simulink model "hybrid_photovoltaic_wind_power_sysytem_grid"  (R2024b)
settings: Solver=ode45  StartTime=0.0  StopTime=1  RelTol=1e-3  EnableMultiTasking=on
undefined symbols (not defined in the file): DiscIntNeverNeededParam, find_system
libraries: powerlib_extras x39, spsThreePhaseVIMeasurementLib x12, spsSeriesRLCBranchLib x5, spsDiodeLib x4, spsUniversalBridgeLib x4, simulink_extras x4, spsThreePhaseBreakerLib x3, spsLoadFlowBusLib x3, spsVoltageMeasurementLib x2, slpidlib x2, spsThreePhaseSeriesRLCLoadLib x2, spsThreePhaseTransformerInductanceMatrixTypeTwoWindingsLib x2
(part 2 of 4)

== system hybrid_photovoltaic_wind_power_sysytem_grid/Hybrid Photovoltaic and Wind power system/VSC1 Control/Current Regulator ==
  note: For Ltot >> Rtot :
  note: (Vq_prim - Vq_conv) ~ = - Id * Ltot
  note: (Vd_prim - Vd_conv) ~= + Iq * Ltot
  note: Ltot = Lxfo + Lchoke
      | Rtot = Rxfo + Rchoke
  note: Id positive --> The converter generates active power ("Inverter mode") = Active Power P positive
  note: Iq positive --> The converter absorbs reactive power ("Inductive mode") = Reactive Power Q negative
  note: Sign Convention: Current going out of the converter = positive current
  note: Current Regulator
      | (with feedforward)
  note: Vq_mes + Id*L + Iq*R + deriv(Iq)*L= Vq_conv
  note: Vd_mes + Id*R - Iq*L + deriv(Id)*L= Vd_conv
  note: harmonic filter neglected
  VdVq_mes : Inport  PortDimensions=2
  IdIq_mes : Inport  Port=2  PortDimensions=2
  IdIq_ref : Inport  Port=3  PortDimensions=2
  Add1 : Sum  Inputs=++-
  Add2 : Sum
  Add3 : Sum  Inputs=+++
  Demux : Demux  Outputs=2
  Demux1 : Demux  Outputs=2
  Ltot_pu1 : Gain  Gain=Ltot_pu  SaturateOnIntegerOverflow=on  OutDataTypeStr=Inherit: Same as input  ParamDataTypeStr=Inherit: Same as input
  Ltot_pu2 : Gain  Gain=Ltot_pu  SaturateOnIntegerOverflow=on  OutDataTypeStr=Inherit: Same as input  ParamDataTypeStr=Inherit: Same as input
  Mux : Mux  Inputs=2
  PI : slpidlib/PID Controller  Controller=PI  Form=Parallel  TimeDomain=Discrete-time  UseExternalTs=off  SampleTime=Ts  IntegratorMethod=Forward Euler  FilterMethod=Forward Euler  ControllerParametersSource=internal  P=Kp_Ireg  I=Ki_Ireg  UseKiTs=off  D=0  UseExternalDerivativeSource=off  N=100  UseFilter=on  TunerSelectOption=Transfer Function Based (PID Tuner App)  InitialConditionSource=internal  InitialConditionForIntegrator=0  InitialConditionForFilter=0  DifferentiatorICPrevScaledInput=0  ExternalReset=none  TrackingMode=off  Kt=1  LimitOutput=on  SatLimitsSource=internal  UpperSaturationLimit=2  LowerSaturationLimit=-2  LinearizeAsGain=off  AntiWindupMode=none  Kb=1  LimitIntegrator=off  UpperIntegratorSaturationLimit=inf  LowerIntegratorSaturationLimit=-inf  POutMin=[]  POutMax=[]  IOutMin=[]  IOutMax=[]  DOutMin=[]  DOutMax=[]  NOutMin=[]  NOutMax=[]  SumOutMin=[]  SumOutMax=[]  SaturationOutMin=[]  SaturationOutMax=[]  PParamMin=[]  PParamMax=[]  IParamMin=[]  IParamMax=[]  DParamMin=[]  DParamMax=[]  NParamMin=[]  NParamMax=[]  KbParamMin=[]  KbParamMax=[]  KtParamMin=[]  KtParamMax=[]  KbOutMin=[]  KbOutMax=[]  KtOutMin=[]  KtOutMax=[]  IntegratorOutMin=[]  IntegratorOutMax=[]  FilterOutMin=[]  FilterOutMax=[]  SumI1OutMin=[]  SumI1OutMax=[]  SumI2OutMin=[]  SumI2OutMax=[]  SumI3OutMin=[]  SumI3OutMax=[]  SumI4OutMin=[]  SumI4OutMax=[]  SumDOutMin=[]  SumDOutMax=[]  DifferentiatorOutMin=[]  DifferentiatorOutMax=[]  FilterDiffOutCoefMin=[]  FilterDiffOutCoefMax=[]  ReciprocalOutMin=[]  ReciprocalOutMax=[]  SumDenOutMin=[]  SumDenOutMax=[]  SumNumOutMin=[]  SumNumOutMax=[]  DivideOutMin=[]  DivideOutMax=[]  UdiffTsProdOutMin=[]  UdiffTsProdOutMax=[]  NTsProdOutMin=[]  NTsProdOutMax=[]  UintegralTsProdOutMin=[]  UintegralTsProdOutMax=[]  UngainTsProdOutMin=[]  UngainTsProdOutMax=[]  ClampingZeroOutDataTypeStr=Inherit: Inherit via back propagation  ClampingZeroOutMin=[]  ClampingZeroOutMax=[]  FilterDenConstantOutDataTypeStr=Inherit: Inherit via back propagation  FilterDenConstantOutMin=[]  FilterDenConstantOutMax=[]  PCopyOutDataTypeStr=Inherit: Inherit via back propagation  PCopyOutMin=[]  PCopyOutMax=[]  NCopyOutDataTypeStr=Inherit: Inherit via back propagation  NCopyOutMin=[]  NCopyOutMax=[]  IntegratorContinuousStateAttributes=''  IntegratorStateMustResolveToSignalObject=off  IntegratorRTWStateStorageClass=Auto  FilterContinuousStateAttributes=''  FilterStateMustResolveToSignalObject=off  FilterRTWStateStorageClass=Auto  ParallelPVariant=InternalParameters  IdealPVariant=Disabled  IVariant=InternalParameters  DVariant=Disabled  IntegratorVariant=Discrete  SatVariant=Enabled  AWVariant=Passthrough  PCopyVariant=Disabled  TRVariant=Disabled  FdbkBlocksVariant=Forward  IdealPFdbkVariant=Disabled  SatFdbkVariant=Disabled  DerivativeFilterVariant=Disabled  NVariant=Disabled  NCopyVariant=Disabled_SignalSpec  FilterICVariant=Disabled  IntegratorICVariant=InternalICs  ExternalResetVariant=Disabled  TRSumVariant=Passthrough  SumFdbkVariant=Disabled  SumVariant=Sum_PI  TsampFilterVariant=InternalTs  TsampNgainVariant=Passthrough  TsampIntegralVariant=Disabled_SignalSpec  ExternalSaturationOutDataTypeStr=Inherit: Same as second input  DerivativeSourceVariant=Disabled  PreIntVariant=InternalPreInt
  PI_Ireg1 : Scope
  Rtot_pu1 : Gain  Gain=Rtot_pu  SaturateOnIntegerOverflow=on  OutDataTypeStr=Inherit: Same as input  ParamDataTypeStr=Inherit: Same as input
  Rtot_pu5 : Gain  Gain=Rtot_pu  SaturateOnIntegerOverflow=on  OutDataTypeStr=Inherit: Same as input  ParamDataTypeStr=Inherit: Same as input
  Saturation : Saturate  UpperLimit=2  LowerLimit=-2
  Sum : Sum  Inputs=|-+
  VdVq_conv : Outport
  wires:
  Add3/1 -> Mux/2
  Demux/2 -> Add3/1
  Add1/1 -> Mux/1  "Feedforward"
  Ltot_pu2/1 -> Add3/3
  Rtot_pu5/1 -> Add3/2
  Demux1/2 -> Rtot_pu5/1, Ltot_pu1/1
  Ltot_pu1/1 -> Add1/3
  Demux1/1 -> Ltot_pu2/1, Rtot_pu1/1
  Rtot_pu1/1 -> Add1/2
  Demux/1 -> Add1/1
  VdVq_mes/1 -> Demux/1
  Saturation/1 -> VdVq_conv/1
  Add2/1 -> Saturation/1
  IdIq_mes/1 -> Sum/1
  IdIq_ref/1 -> Demux1/1, Sum/2
  Sum/1 -> PI/1
  PI/1 -> Add2/1  "PI"
  Mux/1 -> Add2/2, PI_Ireg1/1

== system hybrid_photovoltaic_wind_power_sysytem_grid/Hybrid Photovoltaic and Wind power system/VSC1 Control/PLL & Measurements ==
  Vabc_prim : Inport
  Iabc_prim : Inport  Port=2
  PLL : powerlib_extras/Discrete  Control Blocks/Discrete 3-phase PLL  Fmin=45  Par_Init="[-0.57  Fnom]"  ParK=[60 1400]  Ts=Ts  AGC=off
  Selector1 : Selector  InputPortWidth=3  IndexOptions=Index vector (dialog)  Indices=[1 2]  OutputSizes=1
  Selector2 : Selector  InputPortWidth=3  IndexOptions=Index vector (dialog)  Indices=[1 2]  OutputSizes=1
  Terminator : Terminator
  V->pu : Gain  Gain=1/(Vnom_prim*sqrt(2)/sqrt(3))  SaturateOnIntegerOverflow=on  OutDataTypeStr=Inherit: Same as input  ParamDataTypeStr=Inherit: Same as input
  V->pu1 : Gain  Gain=Vnom_prim*sqrt(3)/Pnom/sqrt(2)  SaturateOnIntegerOverflow=on  OutDataTypeStr=Inherit: Same as input  ParamDataTypeStr=Inherit: Same as input
  abc_to_dq0 Transformation1 : powerlib_extras/Measurements/abc_to_dq0 Transformation
  abc_to_dq0 Transformation2 : powerlib_extras/Measurements/abc_to_dq0 Transformation
  wt : Outport
  VdVq_prim : Outport  Port=2
  IdIq_prim : Outport  Port=3
  wires:
  PLL/1 -> Terminator/1
  PLL/3 -> abc_to_dq0 Transformation1/2, abc_to_dq0 Transformation2/2
  Selector1/1 -> IdIq_prim/1
  Selector2/1 -> VdVq_prim/1
  abc_to_dq0 Transformation1/1 -> Selector2/1
  Iabc_prim/1 -> V->pu1/1
  Vabc_prim/1 -> V->pu/1
  PLL/2 -> wt/1
  abc_to_dq0 Transformation2/1 -> Selector1/1
  V->pu/1 -> abc_to_dq0 Transformation1/1, PLL/1
  V->pu1/1 -> abc_to_dq0 Transformation2/1

== system hybrid_photovoltaic_wind_power_sysytem_grid/Hybrid Photovoltaic and Wind power system/VSC1 Control/Uabc_ref Generation max (m) = 1 ==
  note: (Correction for delai of Ts_Control)
  note: (Correction for transformer
      |  D1 connection)
  wt : Inport
  VdVq_conv : Inport  Port=2
  Add1 : Sum  Inputs=++++
  Add2 : Sum
  Complex to Magnitude-Angle : ComplexToMagnitudeAngle
  Constant : Constant  Value=-pi/6
  Constant1 : Constant  Value=Vnom_dc
  Constant2 : Constant  Value="[ 0  -2*pi/3  2*pi/3  ]"
  Constant3 : Constant  Value=Vnom_sec*sqrt(2)/sqrt(3)
  Constant4 : Constant  Value=Ts*Fnom*(2*pi)
  Demux1 : Demux  Outputs=2
  Gain1 : Gain  Gain=1/2
  Product : Product  Inputs=*/  RndMeth=Zero
  Product1 : Product  Inputs=*/  RndMeth=Zero
  Product2 : Product  Inputs=**  RndMeth=Zero
  Real-Imag to Complex : RealImagToComplex
  Saturation : Saturate  UpperLimit=1  LowerLimit=0
  Trigonometric Function : Trigonometry
  Uabc_ref : Outport
  tag scope: m=global
  wires:
  Constant4/1 -> Add1/4
  wt/1 -> Add1/1
  Product2/1 -> Uabc_ref/1
  Trigonometric Function/1 -> Product2/2
  Saturation/1 -> Product2/1, [m]
  Add2/1 -> Trigonometric Function/1
  Add1/1 -> Add2/2
  Complex to Magnitude-Angle/2 -> Add2/1
  Product/1 -> Product1/2
  Constant3/1 -> Product/2
  Constant/1 -> Add1/3
  Constant2/1 -> Add1/2
  Demux1/2 -> Real-Imag to Complex/2
  Demux1/1 -> Real-Imag to Complex/1
  Real-Imag to Complex/1 -> Complex to Magnitude-Angle/1
  Gain1/1 -> Product/1
  Product1/1 -> Demux1/1
  VdVq_conv/1 -> Product1/1
  Constant1/1 -> Gain1/1
  Complex to Magnitude-Angle/1 -> Saturation/1

== system hybrid_photovoltaic_wind_power_sysytem_grid/Hybrid Photovoltaic and Wind power system/VSC1 Control/VDC Regulator ==
  Vdc_mes : Inport  PortDimensions=1
  Vdc_ref : Inport  Port=2  PortDimensions=1
  PI : slpidlib/PID Controller  Controller=PI  Form=Parallel  TimeDomain=Discrete-time  UseExternalTs=off  SampleTime=Ts  IntegratorMethod=Trapezoidal  FilterMethod=Forward Euler  ControllerParametersSource=internal  P=Kp_VDCreg  I=Ki_VDCreg  UseKiTs=off  D=0  UseExternalDerivativeSource=off  N=100  UseFilter=on  TunerSelectOption=Transfer Function Based (PID Tuner App)  InitialConditionSource=internal  InitialConditionForIntegrator=0  InitialConditionForFilter=0  DifferentiatorICPrevScaledInput=0  ExternalReset=none  TrackingMode=off  Kt=1  LimitOutput=on  SatLimitsSource=internal  UpperSaturationLimit=1.5  LowerSaturationLimit=-1.5  LinearizeAsGain=off  AntiWindupMode=none  Kb=1  LimitIntegrator=off  UpperIntegratorSaturationLimit=inf  LowerIntegratorSaturationLimit=-inf  POutMin=[]  POutMax=[]  IOutMin=[]  IOutMax=[]  DOutMin=[]  DOutMax=[]  NOutMin=[]  NOutMax=[]  SumOutMin=[]  SumOutMax=[]  SaturationOutMin=[]  SaturationOutMax=[]  PParamMin=[]  PParamMax=[]  IParamMin=[]  IParamMax=[]  DParamMin=[]  DParamMax=[]  NParamMin=[]  NParamMax=[]  KbParamMin=[]  KbParamMax=[]  KtParamMin=[]  KtParamMax=[]  KbOutMin=[]  KbOutMax=[]  KtOutMin=[]  KtOutMax=[]  IntegratorOutMin=[]  IntegratorOutMax=[]  FilterOutMin=[]  FilterOutMax=[]  SumI1OutMin=[]  SumI1OutMax=[]  SumI2OutMin=[]  SumI2OutMax=[]  SumI3OutMin=[]  SumI3OutMax=[]  SumI4OutMin=[]  SumI4OutMax=[]  SumDOutMin=[]  SumDOutMax=[]  DifferentiatorOutMin=[]  DifferentiatorOutMax=[]  FilterDiffOutCoefMin=[]  FilterDiffOutCoefMax=[]  ReciprocalOutMin=[]  ReciprocalOutMax=[]  SumDenOutMin=[]  SumDenOutMax=[]  SumNumOutMin=[]  SumNumOutMax=[]  DivideOutMin=[]  DivideOutMax=[]  UdiffTsProdOutMin=[]  UdiffTsProdOutMax=[]  NTsProdOutMin=[]  NTsProdOutMax=[]  UintegralTsProdOutMin=[]  UintegralTsProdOutMax=[]  UngainTsProdOutMin=[]  UngainTsProdOutMax=[]  ClampingZeroOutDataTypeStr=Inherit: Inherit via back propagation  ClampingZeroOutMin=[]  ClampingZeroOutMax=[]  FilterDenConstantOutDataTypeStr=Inherit: Inherit via back propagation  FilterDenConstantOutMin=[]  FilterDenConstantOutMax=[]  PCopyOutDataTypeStr=Inherit: Inherit via back propagation  PCopyOutMin=[]  PCopyOutMax=[]  NCopyOutDataTypeStr=Inherit: Inherit via back propagation  NCopyOutMin=[]  NCopyOutMax=[]  IntegratorContinuousStateAttributes=''  IntegratorStateMustResolveToSignalObject=off  IntegratorRTWStateStorageClass=Auto  FilterContinuousStateAttributes=''  FilterStateMustResolveToSignalObject=off  FilterRTWStateStorageClass=Auto  ParallelPVariant=InternalParameters  IdealPVariant=Disabled  IVariant=InternalParameters  DVariant=Disabled  IntegratorVariant=Discrete  SatVariant=Enabled  AWVariant=Passthrough  PCopyVariant=Disabled  TRVariant=Disabled  FdbkBlocksVariant=Forward  IdealPFdbkVariant=Disabled  SatFdbkVariant=Disabled  DerivativeFilterVariant=Disabled  NVariant=Disabled  NCopyVariant=Disabled_SignalSpec  FilterICVariant=Disabled  IntegratorICVariant=InternalICs  ExternalResetVariant=Disabled  TRSumVariant=Passthrough  SumFdbkVariant=Disabled  SumVariant=Sum_PI  TsampFilterVariant=InternalTs  TsampNgainVariant=Passthrough  TsampIntegralVariant=Disabled_SignalSpec  ExternalSaturationOutDataTypeStr=Inherit: Same as second input  DerivativeSourceVariant=Disabled  PreIntVariant=InternalPreInt
  Rtot_pu3 : Gain  Gain=1/Vnom_dc  SaturateOnIntegerOverflow=on  OutDataTypeStr=Inherit: Same as input  ParamDataTypeStr=Inherit: Same as input
  Sum : Sum  Inputs=|+-
  Id_ref : Outport  SampleTime=Ts  InitialOutput=0
  wires:
  PI/1 -> Id_ref/1
  Rtot_pu3/1 -> PI/1
  Vdc_ref/1 -> Sum/2
  Vdc_mes/1 -> Sum/1
  Sum/1 -> Rtot_pu3/1

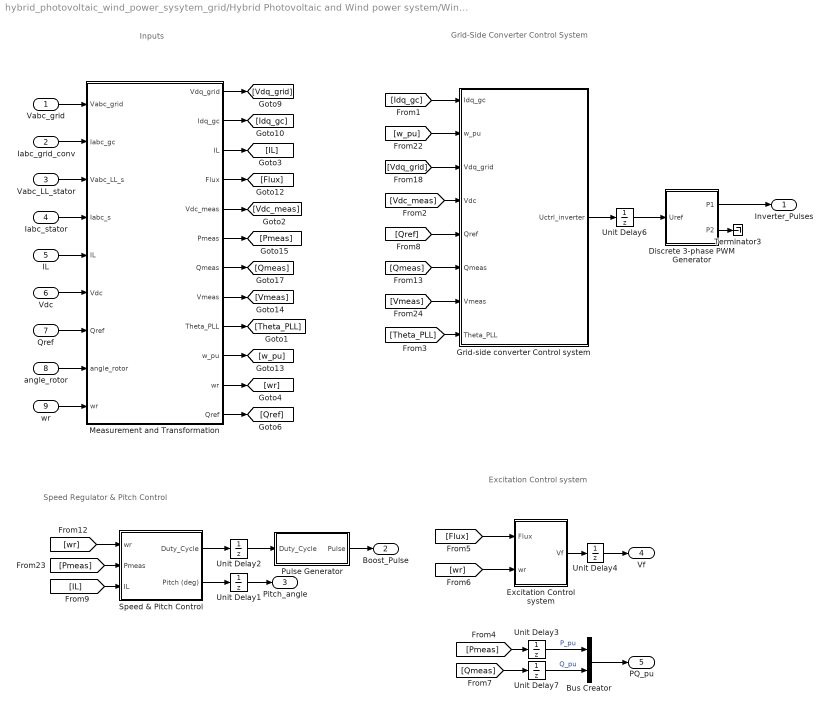
== system hybrid_photovoltaic_wind_power_sysytem_grid/Hybrid Photovoltaic and Wind power system/Wind Turbine Type 4/Control ==
  note: Inputs
  note: Grid-Side Converter
      | Control System
  note: Speed Regulator & Pitch Control
  note: Excitation
      | Control system
  Vabc_grid : Inport
  Iabc_grid_conv : Inport  Port=2
  Vabc_LL_stator : Inport  Port=3
  Iabc_stator : Inport  Port=4
  IL : Inport  Port=5
  Vdc : Inport  Port=6
  Qref : Inport  Port=7
  angle_rotor : Inport  Port=8
  wr : Inport  Port=9
  Bus Creator : BusCreator  Inputs=2
  Discrete 3-phase PWM Generator : Subsystem  DialogController=POWERSYS.PowerSysDialog  mask(Discrete 3-phase PWM Generator (2- or 3-level)){ModulatorType=2-level, ModulatorMode=Un-synchronized, nF=27, Fc=Freq_PWM, ModulatingSignals=off, m=0.2, Freq=60, Phase=0, Ts=Ts}
      mask prompts: ModulatorType "Type"; ModulatorMode "Mode of operation"; nF "Switching ratio: chopping frequency / output frequency"; Fc "Carrier frequency (Hz):"; ModulatingSignals "Internal generation of modulating signal(s)"; m "Modulation Index:"; Freq "Output voltage frequency (Hz):"; Phase "Output voltage phase (degrees):"; Ts "Sample time:"
      mask help:
      | The Discrete 3-phase PWM Generator block generates pulses for carrier-based
      | Pulse Width Modulation (PWM) converters. The block can be used to fire the
      | forced-commuted devices (FETs, GTOs, or IGBTs) of 2-level or 3-level converters
      | using a single  bridge or two bridges connected in twin configuration. Vectorized
      | outputs P1 and P2 contain  either 6 pulses (2-level) or 12 pulses (3-level).
      |
      | Use output P1 when operating in single-bridge configuration. The modulating
      | signals can be applied at Input 1 (Uref) and the synchronization signal at input 2 (wt).
      | Look under the mask' of the block to get a description of the pulse pattern.
      mask init:
      | powericon('psbcallbacks',gcb,'Discrete 3-phase PWM Generator');
      | if ModulatorType==1
      |     nPulses=6;
      |     SelectorElements=[1:1:12];
      | else
      |     nPulses=12;
      |  SelectorElements=[1:1:24];
      | end
      | if (ModulatingSignals==1 & ModulatorMode==2),
      |       CmdModulatingSignals=2;
      | else
      |       CmdModulatingSignals=1;
      | end
      | power_initmask();
      mask Help: This block is part of a subset of blocks in the Extras library that does not have documentation associated with it, other than the block mask description.
      mask TypeOptions ModulatorType: 2-level | 3-level
      mask TypeOptions ModulatorMode: Synchronized | Un-synchronized
      mask Callback ModulatorMode: powericon('psbcallbacks',gcb,'Discrete 3-phase PWM Generator',2);
      mask Callback ModulatingSignals: powericon('psbcallbacks',gcb,'Discrete 3-phase PWM Generator',5);
  Excitation Control system : Subsystem
  Grid-side converter Control system : Subsystem
  Measurement and Transformation : Subsystem
  Pulse Generator : Subsystem  mask{Freq_sawtooth=Freq_sawtooth, Ts=Ts}
      mask prompts: Freq_sawtooth "Frequency of the carrier (sawtooth signal) (Hz):"; Ts "Sample time (Ts) (s):"
  Speed & Pitch Control : Subsystem
  Terminator3 : Terminator
  Unit Delay{1..4,6..7} (6 alike) : UnitDelay  SampleTime=Ts  HasFrameUpgradeWarning=on
  Inverter_Pulses : Outport
  Boost_Pulse : Outport  Port=2
  Pitch_angle : Outport  Port=3
  Vf : Outport  Port=4
  PQ_pu : Outport  Port=5
  wires:
  Excitation Control system/1(Vf) -> Unit Delay4/1
  Speed & Pitch Control/2(Pitch (deg)) -> Unit Delay1/1
  [Idq_gc] -> Grid-side converter Control system/1(Idq_gc)
  [w_pu] -> Grid-side converter Control system/2(w_pu)
  [Vdq_grid] -> Grid-side converter Control system/3(Vdq_grid)
  [Vdc_meas] -> Grid-side converter Control system/4(Vdc)
  [Qref] -> Grid-side converter Control system/5(Qref)
  [Qmeas] -> Grid-side converter Control system/6(Qmeas)
  [Vmeas] -> Grid-side converter Control system/7(Vmeas)
  Speed & Pitch Control/1(Duty_Cycle) -> Unit Delay2/1
  [Flux] -> Excitation Control system/1(Flux)
  [wr] -> Excitation Control system/2(wr)
  [Theta_PLL] -> Grid-side converter Control system/8(Theta_PLL)
  Unit Delay2/1 -> Pulse Generator/1(Duty_Cycle)
  Unit Delay1/1 -> Pitch_angle/1
  Unit Delay4/1 -> Vf/1
  Discrete 3-phase PWM Generator/1(P1) -> Inverter_Pulses/1
  Discrete 3-phase PWM Generator/2(P2) -> Terminator3/1
  Grid-side converter Control system/1(Uctrl_inverter) -> Unit Delay6/1
  Pulse Generator/1(Pulse) -> Boost_Pulse/1
  Unit Delay6/1 -> Discrete 3-phase PWM Generator/1(Uref)
  Bus Creator/1 -> PQ_pu/1
  [Pmeas] -> Unit Delay3/1
  [Qmeas] -> Unit Delay7/1
  Unit Delay3/1 -> Bus Creator/1  "P_pu"
  Unit Delay7/1 -> Bus Creator/2  "Q_pu"
  [wr] -> Speed & Pitch Control/1(wr)
  [Pmeas] -> Speed & Pitch Control/2(Pmeas)
  [IL] -> Speed & Pitch Control/3(IL)
  Vabc_grid/1 -> Measurement and Transformation/1(Vabc_grid)
  Iabc_grid_conv/1 -> Measurement and Transformation/2(Iabc_gc)
  Vabc_LL_stator/1 -> Measurement and Transformation/3(Vabc_LL_s)
  Iabc_stator/1 -> Measurement and Transformation/4(Iabc_s)
  IL/1 -> Measurement and Transformation/5(IL)
  Vdc/1 -> Measurement and Transformation/6(Vdc)
  Qref/1 -> Measurement and Transformation/7(Qref)
  angle_rotor/1 -> Measurement and Transformation/8(angle_rotor)
  wr/1 -> Measurement and Transformation/9(wr)
  Measurement and Transformation/1(Vdq_grid) -> [Vdq_grid]
  Measurement and Transformation/2(Idq_gc) -> [Idq_gc]
  Measurement and Transformation/3("IL ") -> [IL]
  Measurement and Transformation/4(Flux) -> [Flux]
  Measurement and Transformation/5(Vdc_meas) -> [Vdc_meas]
  Measurement and Transformation/6(Pmeas) -> [Pmeas]
  Measurement and Transformation/7(Qmeas) -> [Qmeas]
  Measurement and Transformation/8(Vmeas) -> [Vmeas]
  Measurement and Transformation/9(Theta_PLL) -> [Theta_PLL]
  Measurement and Transformation/10(w_pu) -> [w_pu]
  Measurement and Transformation/11("wr ") -> [wr]
  Measurement and Transformation/12("Qref ") -> [Qref]

== system hybrid_photovoltaic_wind_power_sysytem_grid/Hybrid Photovoltaic and Wind power system/Wind Turbine Type 4/Drive Train ==
  note: Wind turbine drive train based on a 2-masse model
  note: Turbine
  note: Shaft
  T_wt (pu) : Inport
  Generator speed (pu) : Inport  Port=2
  1_2H_WT : Gain  Gain=1/(2*H_WT)  SaturateOnIntegerOverflow=on  OutDataTypeStr=Inherit: Same as input  ParamDataTypeStr=Inherit: Same as input
  Discrete-Time Integrator : DiscreteIntegrator  InitialCondition=w_wt0  SampleTime=Ts  ICPrevOutput=DiscIntNeverNeededParam  ICPrevScaledInput=DiscIntNeverNeededParam
  Discrete-Time Integrator1 : DiscreteIntegrator  InitialCondition=torque0/Ksh  SampleTime=Ts  ICPrevOutput=DiscIntNeverNeededParam  ICPrevScaledInput=DiscIntNeverNeededParam
  Mutual damping : Gain  Gain=D_mutual  SaturateOnIntegerOverflow=on  OutDataTypeStr=Inherit: Same as input  ParamDataTypeStr=Inherit: Same as input
  Stiffness : Gain  Gain=Ksh  SaturateOnIntegerOverflow=on  OutDataTypeStr=Inherit: Same as input  ParamDataTypeStr=Inherit: Same as input
  Sum : Sum  Inputs=+-  InputSameDT=on  SaturateOnIntegerOverflow=on  OutDataTypeStr=Inherit: Same as first input
  Sum1 : Sum  Inputs=+-  InputSameDT=on  SaturateOnIntegerOverflow=on  OutDataTypeStr=Inherit: Same as first input
  Sum2 : Sum  InputSameDT=on  SaturateOnIntegerOverflow=on  OutDataTypeStr=Inherit: Same as first input
  wbase : Gain  Gain=wbase  SaturateOnIntegerOverflow=on  OutDataTypeStr=Inherit: Same as input  ParamDataTypeStr=Inherit: Same as input
  W_wt (pu) : Outport
  T_shaft (pu) : Outport  Port=2
  wires:
  T_wt (pu)/1 -> Sum/1
  Sum2/1 -> T_shaft (pu)/1, Sum/2
  Mutual damping/1 -> Sum2/2
  Sum1/1 -> Mutual damping/1, wbase/1
  Generator speed (pu)/1 -> Sum1/2
  Discrete-Time Integrator/1 -> W_wt (pu)/1, Sum1/1
  1_2H_WT/1 -> Discrete-Time Integrator/1
  Sum/1 -> 1_2H_WT/1
  Stiffness/1 -> Sum2/1
  Discrete-Time Integrator1/1 -> Stiffness/1
  wbase/1 -> Discrete-Time Integrator1/1

== system hybrid_photovoltaic_wind_power_sysytem_grid/Hybrid Photovoltaic and Wind power system/Wind Turbine Type 4/Wind Turbine ==
  W_wt (pu) : Inport
  Pitch angle (deg) : Inport  Port=2
  Wind speed (m/s) : Inport  Port=3
  ->pu : Gain  Gain=1/Prated
  Avoid div. by zero : Saturate  UpperLimit=inf  LowerLimit=eps
  "Avoid div. by zero " : Saturate  UpperLimit=inf  LowerLimit=eps
  Fcn1 : Fcn  Expr=K1*u[2]/u[1]
  Fcn2 : Fcn  Expr=c1*(c6*u[1] + (-c4 - c3*(2.5 + u[2]) + c2*(1/(u[1] + c7*(2.5 + u[2])) -c8/(1 + (2.5 + u[2])^3)))/exp(c5*(1/(u[1] + c7*(2.5 + u[2])) - c8/(1 + (2.5 + u[2])^3))))
  "K2*Cp*wind^3 " : Fcn  Expr=K2*u[1]^3*u[2]
  Mux : Mux  Inputs=2
  Mux1 : Mux  Inputs=2
  Mux2 : Mux  Inputs=2
  Product2 : Product  Inputs=*/  InputSameDT=on  SaturateOnIntegerOverflow=on  OutDataTypeStr=Inherit: Same as first input
  Tt (pu) : Outport
  wires:
  ->pu/1 -> Product2/1  "power_pu"
  Product2/1 -> Tt (pu)/1
  Wind speed (m/s)/1 -> Avoid div. by zero/1
  Fcn1/1 -> Mux1/1  "lambda"
  Mux1/1 -> Fcn2/1
  Mux/1 -> Fcn1/1
  Fcn2/1 -> Mux2/2  "Cp"
  Mux2/1 -> "K2*Cp*wind^3 "/1
  Pitch angle (deg)/1 -> Mux1/2
  W_wt (pu)/1 -> "Avoid div. by zero "/1
  Avoid div. by zero/1 -> Mux2/1, Mux/1
  "Avoid div. by zero "/1 -> Mux/2, Product2/2
  "K2*Cp*wind^3 "/1 -> ->pu/1

== system hybrid_photovoltaic_wind_power_sysytem_grid/Hybrid Photovoltaic and Wind power system/PV array1/Subsystem1/Subsystem ==
  Isc : Inport
  S : Inport  Port=2
  Tamb : Inport  Port=3
  Tref : Inport  Port=4
  Add : Sum
  Add1 : Sum
  Constant1 : Constant
  Constant2 : Constant  Value=0.03
  Divide : Product  Inputs=*/
  Product{,1..3} (4 alike) : Product  RndMeth=Zero
  Sref : Constant  Value=1000
  Subtract : Sum  Inputs=+-
  a : Constant  Value=0.0025
  Isc' : Outport
  wires:
  Add1/1 -> Subtract/1
  Tamb/1 -> Add1/2
  Product3/1 -> Add1/1
  Constant2/1 -> Product3/2
  Tref/1 -> Subtract/2
  Divide/1 -> Isc'/1
  Sref/1 -> Divide/2
  Product2/1 -> Divide/1
  Add/1 -> Product2/2
  Product1/1 -> Product2/1
  S/1 -> Product1/2, Product3/1
  Isc/1 -> Product1/1
  Product/1 -> Add/1
  Constant1/1 -> Add/2
  a/1 -> Product/1
  Subtract/1 -> Product/2

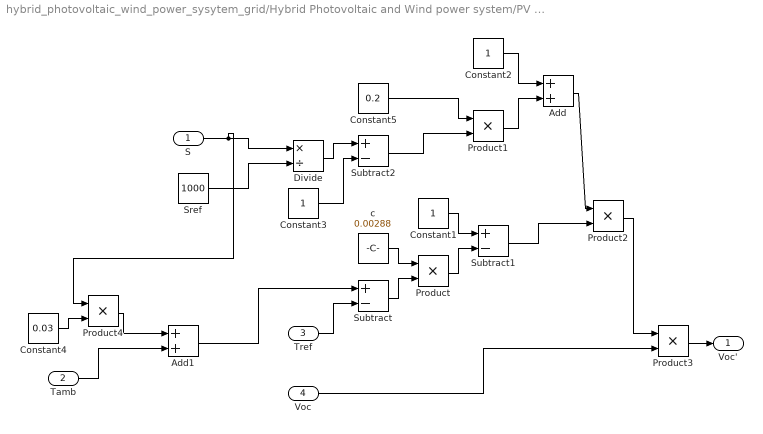
== system hybrid_photovoltaic_wind_power_sysytem_grid/Hybrid Photovoltaic and Wind power system/PV array1/Subsystem1/Subsystem1 ==
  S : Inport
  Tamb : Inport  Port=2
  Tref : Inport  Port=3
  Voc : Inport  Port=4
  Add : Sum
  Add1 : Sum
  Constant1 : Constant
  Constant2 : Constant
  Constant3 : Constant
  Constant4 : Constant  Value=0.03
  Constant5 : Constant  Value=0.2
  Divide : Product  Inputs=*/
  Product{,1..4} (5 alike) : Product  RndMeth=Zero
  Sref : Constant  Value=1000
  Subtract : Sum  Inputs=+-
  Subtract1 : Sum  Inputs=+-
  Subtract2 : Sum  Inputs=+-
  c : Constant  Value=0.00288
  Voc' : Outport
  wires:
  Constant5/1 -> Product1/1
  Add1/1 -> Subtract/1
  Tamb/1 -> Add1/2
  Product4/1 -> Add1/1
  Constant4/1 -> Product4/2
  Constant3/1 -> Subtract2/2
  Divide/1 -> Subtract2/1
  Sref/1 -> Divide/2
  S/1 -> Product4/1, Divide/1
  Product3/1 -> Voc'/1
  Voc/1 -> Product3/2
  Product2/1 -> Product3/1
  Add/1 -> Product2/1
  Subtract1/1 -> Product2/2
  Product1/1 -> Add/2
  Constant2/1 -> Add/1
  Subtract2/1 -> Product1/2
  Product/1 -> Subtract1/2
  Constant1/1 -> Subtract1/1
  Subtract/1 -> Product/2
  c/1 -> Product/1
  Tref/1 -> Subtract/2

== system hybrid_photovoltaic_wind_power_sysytem_grid/Hybrid Photovoltaic and Wind power system/PV array1/Subsystem1/Subsystem2 ==
  Im : Inport
  S : Inport  Port=2
  Tamb : Inport  Port=3
  Tref : Inport  Port=4
  Add : Sum
  Add1 : Sum
  Constant1 : Constant
  Constant2 : Constant  Value=0.03
  Divide : Product  Inputs=*/
  Product{,1..3} (4 alike) : Product  RndMeth=Zero
  Sref : Constant  Value=1000
  Subtract : Sum  Inputs=+-
  a : Constant  Value=0.0025
  Im' : Outport
  wires:
  Add1/1 -> Subtract/1
  Tamb/1 -> Add1/2
  Product3/1 -> Add1/1
  Constant2/1 -> Product3/2
  Tref/1 -> Subtract/2
  Divide/1 -> Im'/1
  Sref/1 -> Divide/2
  Product2/1 -> Divide/1
  Add/1 -> Product2/2
  Product1/1 -> Product2/1
  S/1 -> Product1/2, Product3/1
  Im/1 -> Product1/1
  Product/1 -> Add/1
  Constant1/1 -> Add/2
  a/1 -> Product/1
  Subtract/1 -> Product/2

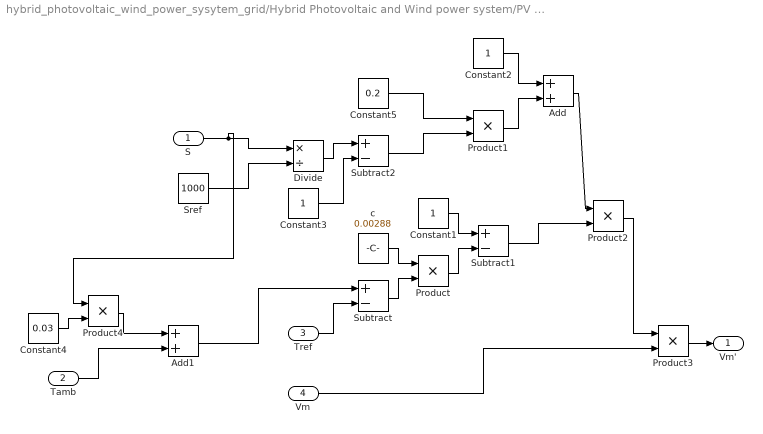
== system hybrid_photovoltaic_wind_power_sysytem_grid/Hybrid Photovoltaic and Wind power system/PV array1/Subsystem1/Subsystem3 ==
  S : Inport
  Tamb : Inport  Port=2
  Tref : Inport  Port=3
  Vm : Inport  Port=4
  Add : Sum
  Add1 : Sum
  Constant1 : Constant
  Constant2 : Constant
  Constant3 : Constant
  Constant4 : Constant  Value=0.03
  Constant5 : Constant  Value=0.2
  Divide : Product  Inputs=*/
  Product{,1..4} (5 alike) : Product  RndMeth=Zero
  Sref : Constant  Value=1000
  Subtract : Sum  Inputs=+-
  Subtract1 : Sum  Inputs=+-
  Subtract2 : Sum  Inputs=+-
  c : Constant  Value=0.00288
  Vm' : Outport
  wires:
  Constant5/1 -> Product1/1
  Add1/1 -> Subtract/1
  Tamb/1 -> Add1/2
  Product4/1 -> Add1/1
  Constant4/1 -> Product4/2
  Constant3/1 -> Subtract2/2
  Divide/1 -> Subtract2/1
  Sref/1 -> Divide/2
  S/1 -> Product4/1, Divide/1
  Product3/1 -> Vm'/1
  Vm/1 -> Product3/2
  Product2/1 -> Product3/1
  Add/1 -> Product2/1
  Subtract1/1 -> Product2/2
  Product1/1 -> Add/2
  Constant2/1 -> Add/1
  Subtract2/1 -> Product1/2
  Product/1 -> Subtract1/2
  Constant1/1 -> Subtract1/1
  Subtract/1 -> Product/2
  c/1 -> Product/1
  Tref/1 -> Subtract/2

== system hybrid_photovoltaic_wind_power_sysytem_grid/Hybrid Photovoltaic and Wind power system/PV array1/Subsystem1/Subsystem5 ==
  C2 : Inport
  Vm : Inport  Port=2
  Voc : Inport  Port=3
  Im : Inport  Port=4
  Isc : Inport  Port=5
  Constant : Constant
  Constant1 : Constant  Value=-1
  Divide : Product  Inputs=*/
  Divide1 : Product  Inputs=*/
  Math Function : Math  SignedPower=on
  Product : Product  RndMeth=Zero
  Product1 : Product  RndMeth=Zero
  Product2 : Product  RndMeth=Zero
  Subtract : Sum  Inputs=+-
  C1 : Outport
  wires:
  Divide/1 -> Subtract/2
  Constant/1 -> Subtract/1
  Isc/1 -> Divide/2
  Im/1 -> Divide/1
  C2/1 -> Product/1
  Voc/1 -> Product/2
  Vm/1 -> Divide1/1
  Product2/1 -> C1/1
  Subtract/1 -> Product2/2
  Math Function/1 -> Product2/1
  Product1/1 -> Math Function/1
  Constant1/1 -> Product1/1
  Divide1/1 -> Product1/2
  Product/1 -> Divide1/2

== system hybrid_photovoltaic_wind_power_sysytem_grid/Hybrid Photovoltaic and Wind power system/PV array1/Subsystem1/Subsystem6 ==
  Im : Inport
  Isc : Inport  Port=2
  Vm : Inport  Port=3
  Voc : Inport  Port=4
  Constant : Constant
  Constant1 : Constant
  Divide : Product  Inputs=*/
  Divide1 : Product  Inputs=*/
  Divide2 : Product  Inputs=*/
  Math Function : Math  Operator=log  SignedPower=on
  Subtract : Sum  Inputs=+-
  Subtract1 : Sum  Inputs=+-
  C2 : Outport
  wires:
  Math Function/1 -> Divide2/2
  Subtract/1 -> Divide2/1
  Subtract1/1 -> Math Function/1
  Isc/1 -> Divide1/2
  Im/1 -> Divide1/1
  Voc/1 -> Divide/2
  Vm/1 -> Divide/1
  Divide2/1 -> C2/1
  Divide1/1 -> Subtract1/2
  Constant1/1 -> Subtract1/1
  Constant/1 -> Subtract/2
  Divide/1 -> Subtract/1

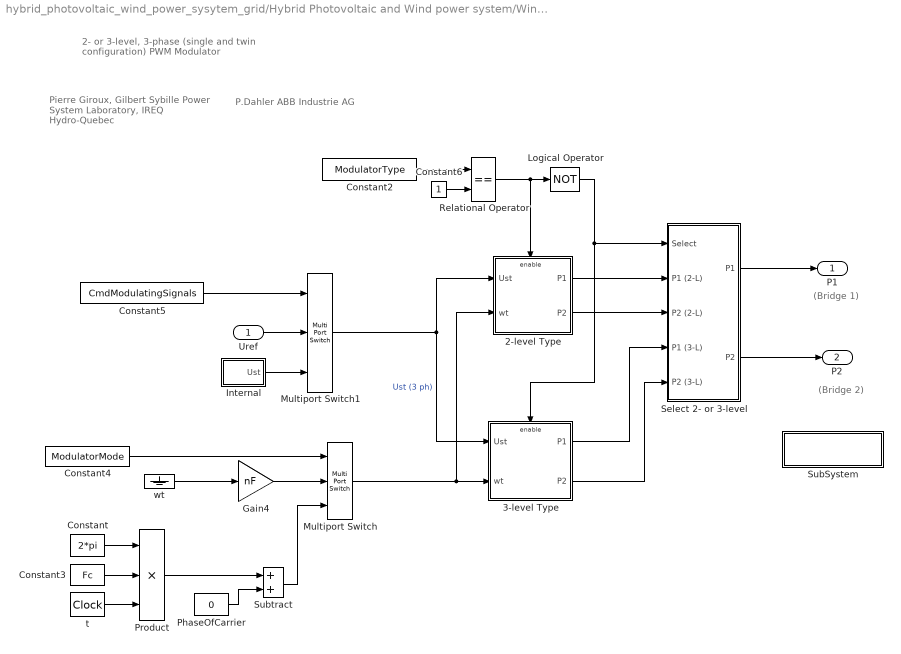
== system hybrid_photovoltaic_wind_power_sysytem_grid/Hybrid Photovoltaic and Wind power system/Wind Turbine Type 4/Control/Discrete 3-phase PWM Generator ==
  note: P.Dahler
      | ABB Industrie AG
  note: (Bridge 1)
  note: (Bridge 2)
  note: 2- or 3-level, 3-phase
      | (single and twin configuration)
      | PWM Modulator
  note: Pierre Giroux, Gilbert Sybille
      | Power System Laboratory, IREQ
      | Hydro-Quebec
  Uref : Inport
  2-level Type : Subsystem  TreatAsAtomicUnit=on
  3-level Type : Subsystem  TreatAsAtomicUnit=on
  Constant : Constant  Value=2*pi
  Constant2 : Constant  Value=ModulatorType
  Constant3 : Constant  Value=Fc
  Constant4 : Constant  Value=ModulatorMode
  Constant5 : Constant  Value=CmdModulatingSignals
  Constant6 : Constant
  Gain4 : Gain  Gain=nF  SaturateOnIntegerOverflow=on  OutDataTypeStr=Inherit: Same as input  ParamDataTypeStr=Inherit: Same as input
  Internal : Subsystem  mask(3-ph signal generator){m=m, Freq=Freq, Phase=Phase, Ts=Ts}
      mask prompts: m "Modulation Index:"; Freq "Output signal frequency (Hz):"; Phase "Output signal phase (degrees):"; Ts "Sample time:"
  Logical Operator : Logic  Operator=NOT
  Multiport Switch : MultiPortSwitch  Inputs=2  SaturateOnIntegerOverflow=off
  Multiport Switch1 : MultiPortSwitch  Inputs=2  SaturateOnIntegerOverflow=off
  PhaseOfCarrier : Constant  Value=0
  Product : Product  Inputs=3  InputSameDT=on  SaturateOnIntegerOverflow=on  OutDataTypeStr=Inherit: Same as first input
  Relational Operator : RelationalOperator  Operator===
  Select 2- or 3-level : Subsystem
  SubSystem : Subsystem
      mask Display: disp('Pulse pattern\ndescription')
  Subtract : Sum
  t : DigitalClock  SampleTime=Ts
  wt : Ground
  P1 : Outport
  P2 : Outport  Port=2
  wires:
  2-level Type/2(P2) -> Select 2- or 3-level/3(P2 (2-L))
  2-level Type/1(P1) -> Select 2- or 3-level/2(P1 (2-L))
  Select 2- or 3-level/1(P1) -> P1/1
  Select 2- or 3-level/2(P2) -> P2/1
  3-level Type/2(P2) -> Select 2- or 3-level/5(P2 (3-L))
  3-level Type/1(P1) -> Select 2- or 3-level/4(P1 (3-L))
  Logical Operator/1 -> Select 2- or 3-level/1(Select), 3-level Type/Enable
  Constant2/1 -> Relational Operator/1
  Relational Operator/1 -> Logical Operator/1, 2-level Type/Enable
  Constant6/1 -> Relational Operator/2
  Multiport Switch1/1 -> 3-level Type/1(Ust), 2-level Type/1(Ust)  "Ust (3 ph)"
  Multiport Switch/1 -> 3-level Type/2(wt), 2-level Type/2(wt)
  Constant/1 -> Product/1
  Constant3/1 -> Product/2
  t/1 -> Product/3
  wt/1 -> Gain4/1
  Constant4/1 -> Multiport Switch/1
  Gain4/1 -> Multiport Switch/2
  Internal/1("Ust ") -> Multiport Switch1/3
  Constant5/1 -> Multiport Switch1/1
  Uref/1 -> Multiport Switch1/2
  PhaseOfCarrier/1 -> Subtract/2
  Product/1 -> Subtract/1
  Subtract/1 -> Multiport Switch/3

== system hybrid_photovoltaic_wind_power_sysytem_grid/Hybrid Photovoltaic and Wind power system/Wind Turbine Type 4/Control/Excitation Control system ==
  Flux : Inport
  wr : Inport  Port=2
  Discrete PI Controller : powerlib_extras/Discrete  Control Blocks/Discrete PI Controller  Kp=Kp_field  Ki=Ki_field  Par_Limits=[1 0]*Vf_limit  Init=init(9)  Ts=Ts
  Divide : Product  Inputs=*/
  Flux_ref : Constant
  "Flux_ref " : Constant
  Sum4 : Sum  Inputs=|+-  InputSameDT=on  SaturateOnIntegerOverflow=on  OutDataTypeStr=Inherit: Same as first input
  Switch : Switch  Threshold=1  SaturateOnIntegerOverflow=off  InputSameDT=off
  avoid division by 0 : Saturate  UpperLimit=inf  LowerLimit=1e-6
  Vf : Outport
  wires:
  Sum4/1 -> Discrete PI Controller/1
  Discrete PI Controller/1 -> Vf/1  "Vf"
  Flux/1 -> Sum4/2  "Flux"
  wr/1 -> Switch/2, avoid division by 0/1
  Flux_ref/1 -> Switch/3
  "Flux_ref "/1 -> Divide/1
  avoid division by 0/1 -> Divide/2
  Divide/1 -> Switch/1
  Switch/1 -> Sum4/1

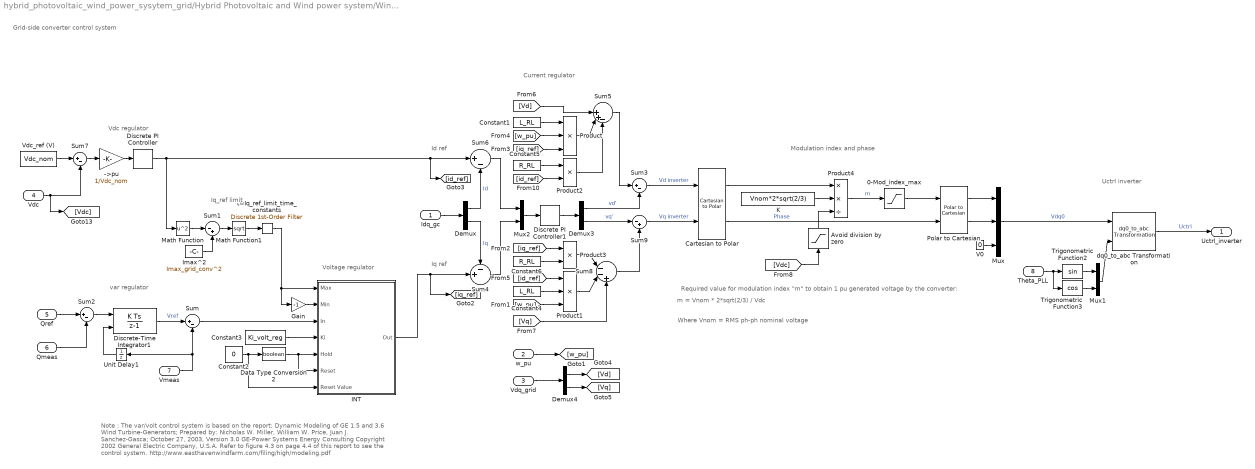
== system hybrid_photovoltaic_wind_power_sysytem_grid/Hybrid Photovoltaic and Wind power system/Wind Turbine Type 4/Control/Grid-side converter Control system ==
  note: Grid-side converter control system
  note: var regulator
  note: Voltage regulator
  note: Vdc regulator
  note: Iq_ref limit
  note: Current regulator
  note: Id ref
  note: Iq ref
  note: Required value for modulation index "m" to obtain 1 pu generated voltage by the converter:
  note: m = Vnom * 2*sqrt(2/3) / Vdc
  note: Where Vnom = RMS ph-ph nominal voltage
  note: Modulation index and phase
  note: Uctrl inverter
  note: Note :
      | The var/volt control system is based on the report:
      | Dynamic Modeling of GE 1.5 and 3.6 Wind Turbine-Generators;
      | Prepared by: Nicholas W. Miller, William W. Price, Juan J. Sanchez-Gasca;
      | October 27, 2003, Version 3.0
      | GE-Power Systems Energy Consulting
      | Copyright 2002 General Electric Company, U.S.A.
      |
      | Refer to figure 4.3 on page 4.4 of this report to see the control system.
      |
      | http://www.easthavenwindfarm.com/filing/high/modeling.pdf
  Idq_gc : Inport
  w_pu : Inport  Port=2
  Vdq_grid : Inport  Port=3
  Vdc : Inport  Port=4
  Qref : Inport  Port=5
  Qmeas : Inport  Port=6
  Vmeas : Inport  Port=7
  Theta_PLL : Inport  Port=8
  ->pu : Gain  Gain=1/Vdc_nom
  0-Mod_index_max : Saturate  UpperLimit=Mod_index_max  LowerLimit=0
  Avoid division by zero : Saturate  UpperLimit=1e6  LowerLimit=1e-6
  Cartesian to Polar : simulink_extras/Transformations/Cartesian to Polar
  Constant1 : Constant  Value=L_RL
  Constant2 : Constant  Value=0
  Constant3 : Constant  Value=Ki_volt_reg
  Constant4 : Constant  Value=L_RL
  Constant5 : Constant  Value=R_RL
  Constant6 : Constant  Value=R_RL
  Data Type Conversion2 : DataTypeConversion  OutDataTypeStr=boolean  SaturateOnIntegerOverflow=off  RndMeth=Floor
  Demux : Demux  Outputs=2
      settings: DisplayOption=none
  Demux3 : Demux  Outputs=2
      settings: DisplayOption=none
  Demux4 : Demux  Outputs=2
      settings: DisplayOption=none
  Discrete PI Controller : powerlib_extras/Discrete  Control Blocks/Discrete PI Controller  Kp=Kp_dc  Ki=Ki_dc  Par_Limits=[1 -1]*Imax_grid_conv  Init=0  Ts=Ts
  Discrete PI Controller1 : powerlib_extras/Discrete  Control Blocks/Discrete PI Controller  Kp=Kp_grid_side_cur_reg  Ki=Ki_grid_side_cur_reg  Par_Limits=[1 -1]*Current_reg_output_limit  Init=0  Ts=Ts
  Discrete-Time Integrator1 : DiscreteIntegrator  gainval=Ki_var_reg  InitialConditionSource=external  InitialCondition=1  SampleTime=Ts  LimitOutput=on  UpperSaturationLimit=Var_reg_output_hi_limit  LowerSaturationLimit=Var_reg_output_low_limit  ICPrevOutput=DiscIntNeverNeededParam  ICPrevScaledInput=DiscIntNeverNeededParam
  Gain : Gain  Gain=-1  SaturateOnIntegerOverflow=on  OutDataTypeStr=Inherit: Same as input  ParamDataTypeStr=Inherit: Same as input
  INT : Subsystem  mask(Integrator  With  External  Dynamic  Limits (Discrete)){}
      mask Display: disp('Discrete-Time\n(Trapezoidal)\nIntegrator\n ')
  Imax^2 : Constant  Value=Imax_grid_conv^2
  K : Constant  Value=Vnom*2*sqrt(2/3)
  Math Function : Math  Operator=square  SignedPower=on
  Math Function1 : Math  Operator=sqrt  SignedPower=on
  Mux : Mux  Inputs=3
  Mux1 : Mux  Inputs=2
  Mux2 : Mux  Inputs=2
  Polar to Cartesian : simulink_extras/Transformations/Polar to Cartesian
  Product : Product  Inputs=3  InputSameDT=on  SaturateOnIntegerOverflow=on  OutDataTypeStr=Inherit: Same as first input
  Product1 : Product  Inputs=3  InputSameDT=on  SaturateOnIntegerOverflow=on  OutDataTypeStr=Inherit: Same as first input
  Product2 : Product  InputSameDT=on  SaturateOnIntegerOverflow=on  OutDataTypeStr=Inherit: Same as first input
  Product3 : Product  InputSameDT=on  SaturateOnIntegerOverflow=on  OutDataTypeStr=Inherit: Same as first input
  Product4 : Product  Inputs=**/  InputSameDT=on  SaturateOnIntegerOverflow=on  OutDataTypeStr=Inherit: Same as first input
  Sum{,2..3,6..7} (5 alike) : Sum  Inputs=|+-  InputSameDT=on  SaturateOnIntegerOverflow=on  OutDataTypeStr=Inherit: Same as first input
  Sum1 : Sum  Inputs=|-+  InputSameDT=on  SaturateOnIntegerOverflow=on  OutDataTypeStr=Inherit: Same as first input
  Sum4 : Sum  Inputs=-+|  InputSameDT=on  SaturateOnIntegerOverflow=on  OutDataTypeStr=Inherit: Same as first input
  Sum5 : Sum  Inputs=||++-  InputSameDT=on  SaturateOnIntegerOverflow=on  OutDataTypeStr=Inherit: Same as first input
  Sum8 : Sum  Inputs=|--+  InputSameDT=on  SaturateOnIntegerOverflow=on  OutDataTypeStr=Inherit: Same as first input
  Sum9 : Sum  Inputs=|-+  InputSameDT=on  SaturateOnIntegerOverflow=on  OutDataTypeStr=Inherit: Same as first input
  Trigonometric Function2 : Trigonometry
  Trigonometric Function3 : Trigonometry  Operator=cos
  Unit Delay1 : UnitDelay  InitialCondition=1  SampleTime=Ts  HasFrameUpgradeWarning=on
  V0 : Constant  Value=0
  Vdc_ref (V) : Constant  Value=Vdc_nom
  dq0_to_abc Transformation : powerlib_extras/Measurements/dq0_to_abc Transformation
  t=Iq_ref_limit_time_constants : powerlib_extras/Discrete  Control Blocks/Discrete 1st-Order Filter  FilterType=Lowpass  Tc=Iq_ref_limit_time_constant  Ts=Ts  Initialize=on  Vac_Init=[0 0 0]  Vdc_Init=Imax_grid_conv  PlotResponse=off  param1=[1 500 0.1]
  Uctrl_inverter : Outport
  wires:
  Vdc/1 -> [Vdc], Sum7/2
  Vdq_grid/1 -> Demux4/1
  Idq_gc/1 -> Demux/1
  Vdc_ref (V)/1 -> Sum7/1
  Sum7/1 -> ->pu/1
  ->pu/1 -> Discrete PI Controller/1
  Discrete PI Controller/1 -> Math Function/1, [id_ref], Sum6/1
  Sum/1 -> INT/3(In)
  Constant2/1 -> Data Type Conversion2/1, INT/7(Reset Value)
  Data Type Conversion2/1 -> INT/5(Hold), INT/6(Reset)
  Gain/1 -> INT/2(Min)
  Constant3/1 -> INT/4(Ki)
  Discrete-Time Integrator1/1 -> Sum/1  "Vref"
  Vmeas/1 -> Unit Delay1/1, Sum/2
  Qmeas/1 -> Sum2/2
  Sum2/1 -> Discrete-Time Integrator1/1
  Unit Delay1/1 -> Discrete-Time Integrator1/2
  Qref/1 -> Sum2/1
  Math Function1/1 -> t=Iq_ref_limit_time_constants/1
  Sum1/1 -> Math Function1/1
  Imax^2/1 -> Sum1/2
  Math Function/1 -> Sum1/1
  t=Iq_ref_limit_time_constants/1 -> INT/1(Max), Gain/1
  Constant4/1 -> Product1/2
  Discrete PI Controller1/1 -> Demux3/1
  Mux2/1 -> Discrete PI Controller1/1
  Constant1/1 -> Product/1
  Demux/2 -> Sum4/1  "Iq"
  Demux/1 -> Sum6/2  "Id"
  Product/1 -> Sum5/2
  Constant5/1 -> Product2/1
  Constant6/1 -> Product3/2
  Product1/1 -> Sum8/2
  Product2/1 -> Sum5/3
  Product3/1 -> Sum8/1
  Sum6/1 -> Mux2/1
  Sum4/1 -> Mux2/2
  [w_pu] -> Product1/3
  [w_pu] -> Product/2
  [iq_ref] -> Product/3
  [id_ref] -> Product2/2
  [iq_ref] -> Product3/1
  [id_ref] -> Product1/1
  Demux3/1 -> Sum3/2  "vd'"
  Demux3/2 -> Sum9/1  "vq'"
  Sum5/1 -> Sum3/1
  Sum8/1 -> Sum9/2
  w_pu/1 -> [w_pu]
  Demux4/1 -> [Vd]
  Demux4/2 -> [Vq]
  [Vq] -> Sum8/3
  [Vd] -> Sum5/1
  INT/1(Out) -> Sum4/2, [iq_ref]
  Product4/1 -> 0-Mod_index_max/1  "m"
  K/1 -> Product4/2
  Avoid division by zero/1 -> Product4/3
  Cartesian to Polar/1 -> Product4/1
  [Vdc] -> Avoid division by zero/1
  Sum3/1 -> Cartesian to Polar/1  "Vd inverter"
  Sum9/1 -> Cartesian to Polar/2  "Vq inverter"
  Theta_PLL/1 -> Trigonometric Function2/1, Trigonometric Function3/1
  Polar to Cartesian/2 -> Mux/2
  Polar to Cartesian/1 -> Mux/1
  V0/1 -> Mux/3
  Trigonometric Function3/1 -> Mux1/2
  Trigonometric Function2/1 -> Mux1/1
  Mux1/1 -> dq0_to_abc Transformation/2
  0-Mod_index_max/1 -> Polar to Cartesian/1
  Cartesian to Polar/2 -> Polar to Cartesian/2  "Phase"
  Mux/1 -> dq0_to_abc Transformation/1  "Vdq0"
  dq0_to_abc Transformation/1 -> Uctrl_inverter/1  "Uctrl"

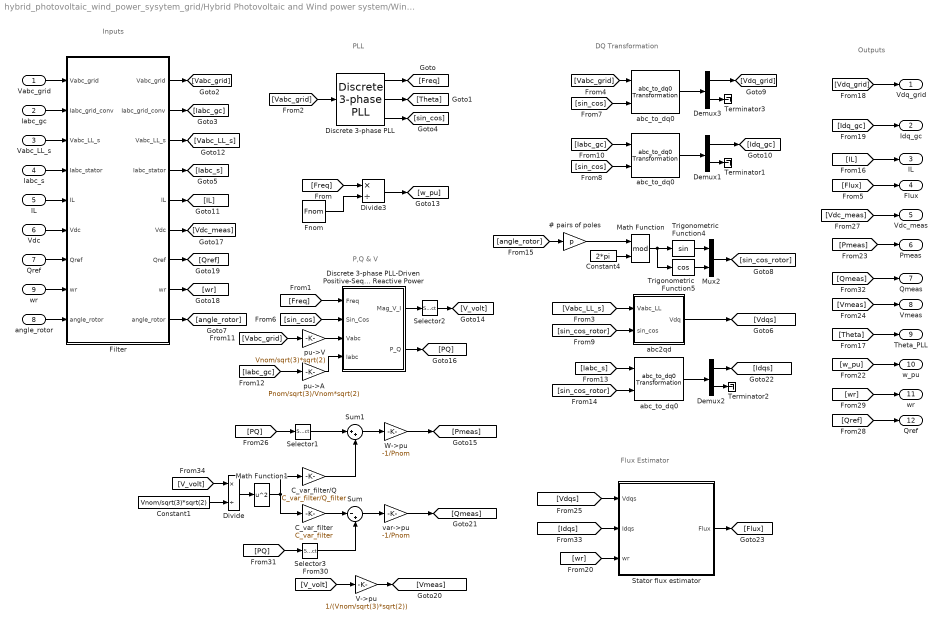
== system hybrid_photovoltaic_wind_power_sysytem_grid/Hybrid Photovoltaic and Wind power system/Wind Turbine Type 4/Control/Measurement and Transformation ==
  note: Flux Estimator
  note: Outputs
  note: PLL
  note: DQ Transformation
  note: P,Q & V
  note: Inputs
  Vabc_grid : Inport
  Iabc_gc : Inport  Port=2
  Vabc_LL_s : Inport  Port=3
  Iabc_s : Inport  Port=4
  IL : Inport  Port=5
  Vdc : Inport  Port=6
  Qref : Inport  Port=7
  angle_rotor : Inport  Port=8
  wr : Inport  Port=9
  "   abc_to_dq0    " : powerlib_extras/Measurements/abc_to_dq0 Transformation
  # pairs of poles : Gain  Gain=p  SaturateOnIntegerOverflow=on  OutDataTypeStr=Inherit: Same as input  ParamDataTypeStr=Inherit: Same as input
  C_var_filter : Gain  Gain=C_var_filter  SaturateOnIntegerOverflow=on  OutDataTypeStr=Inherit: Same as input  ParamDataTypeStr=Inherit: Same as input
  C_var_filter/Q : Gain  Gain=C_var_filter/Q_filter  SaturateOnIntegerOverflow=on  OutDataTypeStr=Inherit: Same as input  ParamDataTypeStr=Inherit: Same as input
  Constant1 : Constant  Value=Vnom/sqrt(3)*sqrt(2)
  Constant4 : Constant  Value=2*pi
  Demux1 : Demux  Outputs=[2 1]
      settings: DisplayOption=none
  Demux2 : Demux  Outputs=[2 1]
      settings: DisplayOption=none
  Demux3 : Demux  Outputs=[2 1]
      settings: DisplayOption=none
  Discrete 3-phase PLL : powerlib_extras/Discrete  Control Blocks/Discrete 3-phase PLL  Fmin=0.75*Fnom  Par_Init=[-45 Fnom]  ParK=[60 1400 1]  Ts=Ts  AGC=off
  Discrete 3-phase PLL-Driven Positive-Sequence Active & Reactive Power : Subsystem  mask(Discrete 3-phase PLL-Driven Positive-Sequence Active & Reactive Power){Finit=Fnom, Fmin=Fnom*45/60, Par_Vinit=[Vnom/sqrt(3)*sqrt(2) 30], Par_Iinit=[Pnom/sqrt(3)/Vnom*sqrt(2) -10], Ts=Ts}
      mask prompts: Finit "Initial frequency (Hz):"; Fmin "Minimum frequency (Hz):"; Par_Vinit "Voltage initial input: [ Mag  Phase(Degrees) ]"; Par_Iinit "Current initial input: [ Mag  Phase(Degrees) ]"; Ts "Sample time:"
      mask help:
      | This discrete block measures the 3-phase active power P and reactive power Q  associated with a periodic set of 3-phase voltages and currents which may contain harmonics. P and Q are calculated by evaluating the fundamental values (positive-sequence) of the input voltages and currents with a running window over one cycle of the specified frequency (port Freq).
      |  Input port "Sin_Cos" (a two-dimension signal) provides the reference frame required for the computation.
      |
      | input 1: must give the frequency of the fundamental (Hz)
      | Input 2: must contain a  [sin(wt)  cos(wt)] two dimension signal , where w is the rotation speed (rad/s) of the reference frame used for the computation..
      | input 3: Vectorized 3-phase  instantaneous voltage (Vabc)
      | input 4: Vectorized 3-phase instantaneous current (Iabc)
      |
      | Output 1: Vector [Mag_V Mag_I] of the fundamental values (Magnitude) of the voltage & current (peak values of the positive-sequence)
      | Output 2: 3-phase PQ measurement vector [P(W) Q (var)] evaluated at the specified frequency. Current flowing into an RL circuit will produce  positive active and reactive powers.
      |
      | For the first cycle of simulation, the outputs are held constant using the values specified by the parameters "Initial input".
      | he value of the parameter "Minimum frequency" is used to determine the buffer size of the "Variable Transport Delay" block found inside this subsystem.
      mask init:
      | power_initmask();
      settings: OpenFcn=power_openblockproxy();
  Divide : Product  Inputs=*/
  Divide3 : Product  Inputs=*/
  Filter : Subsystem  mask{Freq=Freq_filter, Zeta=Zeta_filter, Ts=Ts}
      mask prompts: Freq "Cut-off frequency (Hz):"; Zeta "Damping factor Zeta:"; Ts "Sample time"
  Fnom : Constant  Value=Fnom
  Math Function : Math  Operator=mod  SignedPower=on
  Math Function1 : Math  Operator=square  SignedPower=on
  Mux2 : Mux  Inputs=2
  Selector1 : Selector  InputPortWidth=2  IndexOptions=Index vector (dialog)  Indices=1  OutputSizes=1
  Selector2 : Selector  InputPortWidth=2  IndexOptions=Index vector (dialog)  Indices=1  OutputSizes=1
  Selector3 : Selector  InputPortWidth=2  IndexOptions=Index vector (dialog)  Indices=2  OutputSizes=1
  Stator flux estimator : Subsystem
  Sum : Sum  Inputs=|-+
  Sum1 : Sum  Inputs=|++
  Terminator1 : Terminator
  Terminator2 : Terminator
  Terminator3 : Terminator
  Trigonometric Function4 : Trigonometry
  Trigonometric Function5 : Trigonometry  Operator=cos
  V->pu : Gain  Gain=1/(Vnom/sqrt(3)*sqrt(2))  SaturateOnIntegerOverflow=on  OutDataTypeStr=Inherit: Same as input  ParamDataTypeStr=Inherit: Same as input
  W->pu : Gain  Gain=-1/Pnom  SaturateOnIntegerOverflow=on  OutDataTypeStr=Inherit: Same as input  ParamDataTypeStr=Inherit: Same as input
  abc2qd : Subsystem
  abc_to_dq0 : powerlib_extras/Measurements/abc_to_dq0 Transformation
  "abc_to_dq0  " : powerlib_extras/Measurements/abc_to_dq0 Transformation
  pu->A : Gain  Gain=Pnom/sqrt(3)/Vnom*sqrt(2)  SaturateOnIntegerOverflow=on  OutDataTypeStr=Inherit: Same as input  ParamDataTypeStr=Inherit: Same as input
  pu->V : Gain  Gain=Vnom/sqrt(3)*sqrt(2)  SaturateOnIntegerOverflow=on  OutDataTypeStr=Inherit: Same as input  ParamDataTypeStr=Inherit: Same as input
  "var->pu " : Gain  Gain=-1/Pnom  SaturateOnIntegerOverflow=on  OutDataTypeStr=Inherit: Same as input  ParamDataTypeStr=Inherit: Same as input
  Vdq_grid : Outport
  Idq_gc : Outport  Port=2
  "IL " : Outport  Port=3
  Flux : Outport  Port=4
  Vdc_meas : Outport  Port=5
  Pmeas : Outport  Port=6
  Qmeas : Outport  Port=7
  Vmeas : Outport  Port=8
  Theta_PLL : Outport  Port=9
  w_pu : Outport  Port=10
  "wr " : Outport  Port=11
  "Qref " : Outport  Port=12
  wires:
  Filter/9("angle_rotor ") -> [angle_rotor]
  angle_rotor/1 -> Filter/9(angle_rotor)
  Stator flux estimator/1(Flux) -> [Flux]
  # pairs of poles/1 -> Math Function/1
  Constant4/1 -> Math Function/2
  abc2qd/1(Vdq) -> [Vdqs]
  Trigonometric Function5/1 -> Mux2/2
  Trigonometric Function4/1 -> Mux2/1
  [angle_rotor] -> # pairs of poles/1
  [Vabc_LL_s] -> abc2qd/1(Vabc_LL)
  Math Function/1 -> Trigonometric Function5/1, Trigonometric Function4/1
  [sin_cos_rotor] -> abc2qd/2(sin_cos)
  Mux2/1 -> [sin_cos_rotor]
  Demux2/1 -> [Idqs]
  Demux2/2 -> Terminator2/1
  "   abc_to_dq0    "/1 -> Demux2/1
  [Iabc_s] -> "   abc_to_dq0    "/1
  [sin_cos_rotor] -> "   abc_to_dq0    "/2
  [Vdqs] -> Stator flux estimator/1(Vdqs)
  [Idqs] -> Stator flux estimator/2(Idqs)
  [wr] -> Stator flux estimator/3(wr)
  [Qmeas] -> Qmeas/1
  "var->pu "/1 -> [Qmeas]
  [PQ] -> Selector3/1
  V->pu/1 -> [Vmeas]
  [V_volt] -> V->pu/1
  Selector2/1 -> [V_volt]
  Discrete 3-phase PLL-Driven Positive-Sequence Active & Reactive Power/1(Mag_V_I) -> Selector2/1
  Demux1/2 -> Terminator1/1
  Demux3/1 -> [Vdq_grid]
  Demux3/2 -> Terminator3/1
  "abc_to_dq0  "/1 -> Demux1/1
  abc_to_dq0/1 -> Demux3/1
  Discrete 3-phase PLL/1 -> [Freq]
  Fnom/1 -> Divide3/2
  Divide3/1 -> [w_pu]
  Discrete 3-phase PLL/3 -> [sin_cos]
  pu->V/1 -> Discrete 3-phase PLL-Driven Positive-Sequence Active & Reactive Power/3(Vabc)
  W->pu/1 -> [Pmeas]
  [Freq] -> Divide3/1
  [Freq] -> Discrete 3-phase PLL-Driven Positive-Sequence Active & Reactive Power/1(Freq)
  Discrete 3-phase PLL/2 -> [Theta]
  [Vabc_grid] -> abc_to_dq0/1
  [sin_cos] -> Discrete 3-phase PLL-Driven Positive-Sequence Active & Reactive Power/2(Sin_Cos)
  [sin_cos] -> abc_to_dq0/2
  [sin_cos] -> "abc_to_dq0  "/2
  [Vabc_grid] -> Discrete 3-phase PLL/1
  [Iabc_gc] -> "abc_to_dq0  "/1
  [Theta] -> Theta_PLL/1
  Demux1/1 -> [Idq_gc]
  [Vdq_grid] -> Vdq_grid/1
  [Idq_gc] -> Idq_gc/1
  [w_pu] -> w_pu/1
  [Pmeas] -> Pmeas/1
  [Vmeas] -> Vmeas/1
  pu->A/1 -> Discrete 3-phase PLL-Driven Positive-Sequence Active & Reactive Power/4(Iabc)
  [PQ] -> Selector1/1
  [Vdc_meas] -> Vdc_meas/1
  [Qref] -> "Qref "/1
  [wr] -> "wr "/1
  [Flux] -> Flux/1
  [Vabc_grid] -> pu->V/1
  [Iabc_gc] -> pu->A/1
  Discrete 3-phase PLL-Driven Positive-Sequence Active & Reactive Power/2(P_Q) -> [PQ]
  Vabc_grid/1 -> Filter/1(Vabc_grid)
  Vdc/1 -> Filter/6(Vdc)
  Qref/1 -> Filter/7(Qref)
  wr/1 -> Filter/8(wr)
  Filter/1("Vabc_grid ") -> [Vabc_grid]
  Filter/2("Iabc_grid_conv ") -> [Iabc_gc]
  Filter/4("Iabc_stator ") -> [Iabc_s]
  Filter/6("Vdc ") -> [Vdc_meas]
  Filter/8("wr ") -> [wr]
  Filter/7("Qref ") -> [Qref]
  Iabc_gc/1 -> Filter/2(Iabc_grid_conv)
  Iabc_s/1 -> Filter/4(Iabc_stator)
  Vabc_LL_s/1 -> Filter/3(Vabc_LL_s)
  Filter/3("Vabc_LL_s ") -> [Vabc_LL_s]
  [V_volt] -> Divide/1
  Constant1/1 -> Divide/2
  Divide/1 -> Math Function1/1
  Selector3/1 -> Sum/2
  C_var_filter/1 -> Sum/1
  Sum/1 -> "var->pu "/1
  Math Function1/1 -> C_var_filter/Q/1, C_var_filter/1
  Selector1/1 -> Sum1/1
  C_var_filter/Q/1 -> Sum1/2
  Sum1/1 -> W->pu/1
  IL/1 -> Filter/5(IL)
  Filter/5("IL ") -> [IL]
  [IL] -> "IL "/1

== system hybrid_photovoltaic_wind_power_sysytem_grid/Hybrid Photovoltaic and Wind power system/Wind Turbine Type 4/Control/Pulse Generator ==
  Duty_Cycle : Inport
  Add : Sum  Inputs=-+
  Constant3 : Constant
  Constant4 : Constant  Value=0
  Digital Clock : DigitalClock  SampleTime=Ts
  Divide2 : Product  Inputs=**
  Divide3 : Product  Inputs=**
  Math Function : Math  Operator=mod  SignedPower=on
  Nb_of_samples_by_cycle : Constant  Value=1/Freq_sawtooth/Ts
  Relational Operator1 : RelationalOperator  Operator=>  OutDataTypeStr=boolean  InputSameDT=off
  Rounding Function1 : Rounding  Operator=round
  Switch : Switch  Threshold=0.5  SaturateOnIntegerOverflow=off  InputSameDT=off
  Ts : Constant  Value=Ts
  Pulse : Outport
  wires:
  Math Function/1 -> Relational Operator1/2
  Constant4/1 -> Switch/3
  Constant3/1 -> Switch/1
  Relational Operator1/1 -> Switch/2
  Nb_of_samples_by_cycle/1 -> Rounding Function1/1
  Divide2/1 -> Relational Operator1/1
  Divide3/1 -> Add/2, Math Function/2  "Period_of_cycle"
  Duty_Cycle/1 -> Divide2/1
  Rounding Function1/1 -> Divide3/2  "Nb_of_samples_by_cycle"
  Ts/1 -> Divide3/1, Add/1
  Digital Clock/1 -> Math Function/1
  Add/1 -> Divide2/2
  Switch/1 -> Pulse/1
